simulink model "Simulink_Lab1"  (R2022a)
settings: Solver=VariableStepAuto  StartTime=0.0  StopTime=10.0  RelTol=1e-3
settings Model: Creator=bebawy  LastModifiedBy=bebawy

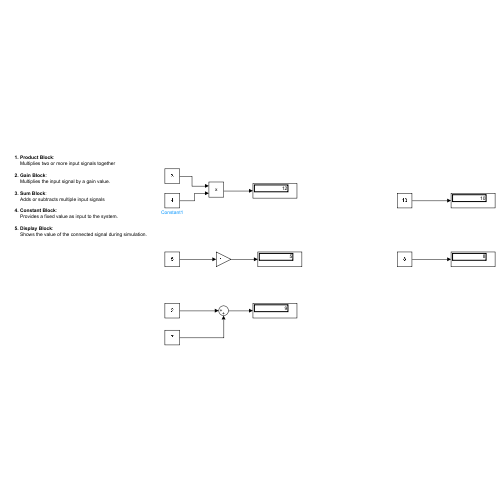
[thumbnail: Simulink's stored preview of the top-level diagram]
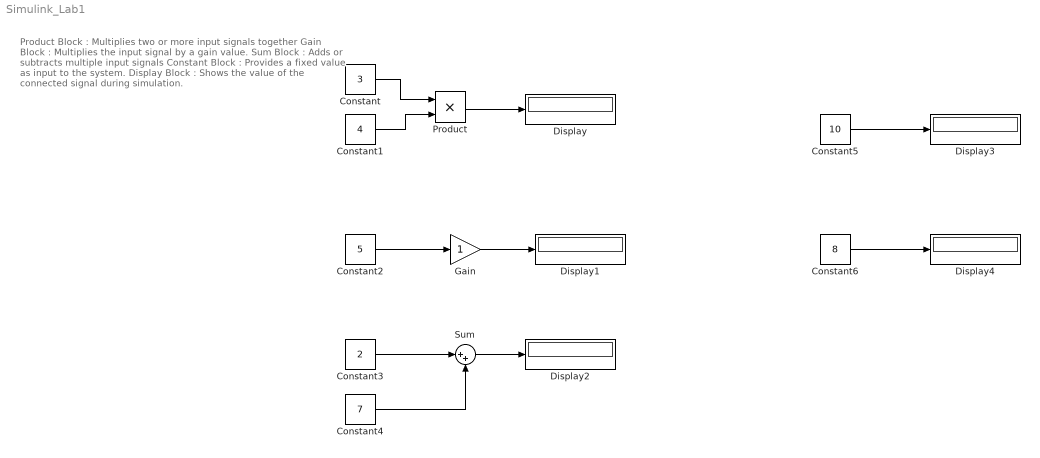
== system Simulink_Lab1 ==
  note: Product Block :
      | Multiplies two or more input signals together
      | Gain Block :
      | Multiplies the input signal by a gain value.
      | Sum Block :
      | Adds or subtracts multiple input signals
      | Constant Block :
      | Provides a fixed value as input to the system.
      | Display Block :
      | Shows the value of the connected signal during simulation.
  Constant : Constant  Value=3
  Constant1 : Constant  Value=4
  Constant2 : Constant  Value=5
  Constant3 : Constant  Value=2
  Constant4 : Constant  Value=7
  Constant5 : Constant  Value=10
  Constant6 : Constant  Value=8
  Display{,1..4} (5 alike) : Display
  Gain : Gain
  Product : Product
  Sum : Sum  Inputs=|++
  wires:
  Product/1 -> Display/1
  Constant/1 -> Product/1
  Constant1/1 -> Product/2
  Constant2/1 -> Gain/1
  Gain/1 -> Display1/1
  Constant3/1 -> Sum/1
  Constant4/1 -> Sum/2
  Sum/1 -> Display2/1
  Constant5/1 -> Display3/1
  Constant6/1 -> Display4/1
